simulink model "slider_mode_controller_kalman_filter_sim_18"  (R2022a)
settings: Solver=ode5  StartTime=0.0  StopTime=700  RelTol=1e-3  EnableMultiTasking=on
undefined symbols (not defined in the file): sim_output_sample_time, sim_r
libraries: simulink x1
settings Model: Creator=wolfgang  LastModifiedBy=Alghisi
settings Model: ModifiedHistory=|
  | Created an adjusted empty Simulink diagram for the lab assignments
  | in the course R0002E
settings SolverCC: AlgebraicLoopSolver=TrustRegion
settings DataIOCC: SaveFormat=Array  SignalLoggingSaveFormat=ModelDataLogs  SaveOutput=off  SignalLogging=off  DSMLogging=off  SaveTime=off  ReturnWorkspaceOutputs=off
settings OptimizationCC: ExpressionDepthLimit=2147483647  LifeSpan=inf
settings DebuggingCC: UnderspecifiedInitializationDetection=Classic  MergeDetectMultiDrivingBlocksExec=none  SolverPrmCheckMsg=warning  FcnCallInpInsideContextMsg=warning  UnconnectedInputMsg=warning  UnconnectedOutputMsg=warning  UnconnectedLineMsg=warning  StateNameClashWarn=warning  SFUnexpectedBacktrackingDiag=warning  SFNoUnconditionalDefaultTransitionDiag=warning  SFExecutionAtInitializationDiag=none  SFMachineParentedDataDiag=warning  ArithmeticOperatorsInVariantConditions=warning
settings HardwareCC: ProdBitPerPointer=32  ProdBitPerSizeT=32  ProdBitPerPtrDiffT=32  ProdLargestAtomicFloat=None  ProdIntDivRoundTo=Undefined  ProdEndianess=Unspecified  ProdWordSize=32  ProdHWDeviceType=32-bit Generic
settings ModelReferenceCC: PropagateSignalLabelsOutOfModel=off
settings SFSimCC: SimUseLocalCustomCode=off  CustomCodeUndefinedFunction=UseInterfaceOnly
settings RTWCC: RTWUseLocalCustomCode=off
settings CodeAppCC: StateflowObjectComments=on
settings GRTTargetCC: TargetLangStandard=C89/C90 (ANSI)
settings ConfigComp: CovMetricSettings=dw  CovSaveCumulativeToWorkspaceVar=on  CovSaveSingleToWorkspaceVar=on  CovExternalEMLEnable=off  CovSFcnEnable=off

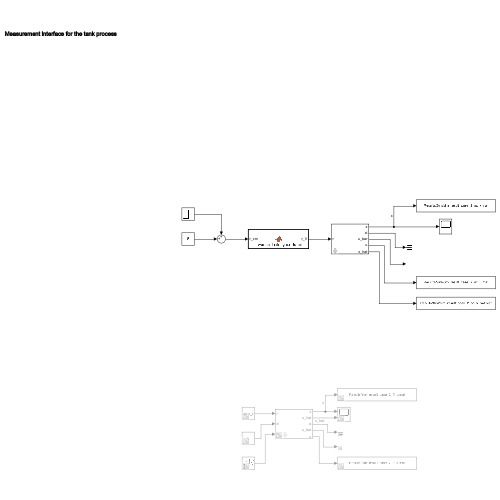
[thumbnail: Simulink's stored preview of the top-level diagram]
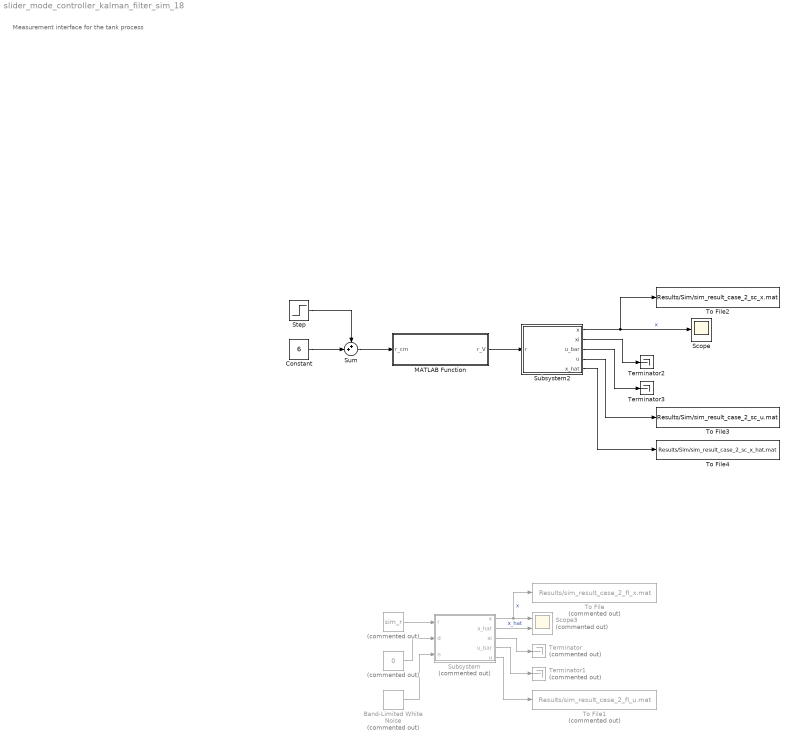
== system slider_mode_controller_kalman_filter_sim_18 ==
  note: Measurement interface for the tank process
  "  " : Constant  Commented=on  Value=0
  "      " : Constant  Commented=on  Value=sim_r
  Band-Limited White Noise : simulink/Sources/Band-Limited White Noise  Commented=on  Cov=0.00001  Ts=0.1  seed=[23341]
  Constant : Constant  Value=6
  MATLAB Function : MATLAB Function  TreatAsAtomicUnit=on
  Scope : Scope
  Scope3 : Scope  Commented=on  NumInputPorts=2
  Step : Step  Time=300  After=2  SampleTime=0
  Subsystem : Subsystem  Commented=on  mask{init_state_param=[8;8], Integrator_gain_param=0.01}
      mask prompts: init_state_param "Initial state"; Integrator_gain_param "Integrator gain"
  Subsystem2 : Subsystem  mask{p1_param=0.1, p2_param=0.2, epsi_param=0.5, mu_param=0.2}
      mask prompts: p1_param "p1"; p2_param "p2"; epsi_param "epsi"; mu_param "mu"
  Sum : Sum  Inputs=++|
  Terminator : Terminator  Commented=on
  Terminator1 : Terminator  Commented=on
  Terminator2 : Terminator
  Terminator3 : Terminator
  To File : ToFile  Commented=on  Filename=Results/sim_result_case_2_fl_x.mat  MatrixName=sim_result_case_2_fl_x  SaveFormat=Timeseries  SampleTime=sim_output_sample_time
  To File1 : ToFile  Commented=on  Filename=Results/sim_result_case_2_fl_u.mat  MatrixName=sim_result_case_2_fl_u  SaveFormat=Timeseries  SampleTime=sim_output_sample_time
  To File2 : ToFile  Filename=Results/Sim/sim_result_case_2_sc_x.mat  MatrixName=sim_result_case_2_sc_x  SaveFormat=Timeseries  SampleTime=0.02
  To File3 : ToFile  Filename=Results/Sim/sim_result_case_2_sc_u.mat  MatrixName=sim_result_case_2_sc_u  SaveFormat=Timeseries  SampleTime=0.02
  To File4 : ToFile  Filename=Results/Sim/sim_result_case_2_sc_x_hat.mat  MatrixName=sim_result_case_2_sc_x_hat  SaveFormat=Timeseries  SampleTime=0.02
  wires:
  Subsystem/2(x_hat) -> Scope3/2  "x_hat"
  "  "/1 -> Subsystem/2(d)
  "      "/1 -> Subsystem/1(r)
  Band-Limited White Noise/1 -> Subsystem/3(n)
  Subsystem/1(x) -> Scope3/1, To File/1  "x"
  Subsystem/3(xi) -> Terminator/1
  Subsystem/4(u_bar) -> Terminator1/1
  Subsystem/5(u) -> To File1/1
  Subsystem2/2(xi) -> Terminator2/1
  MATLAB Function/1(r_V) -> Subsystem2/1(r)
  Subsystem2/3(u_bar) -> Terminator3/1
  Subsystem2/4(u) -> To File3/1
  Subsystem2/1(x) -> Scope/1, To File2/1  "x"
  Constant/1 -> Sum/2
  Sum/1 -> MATLAB Function/1(r_cm)
  Step/1 -> Sum/1
  Subsystem2/5(x_hat) -> To File4/1

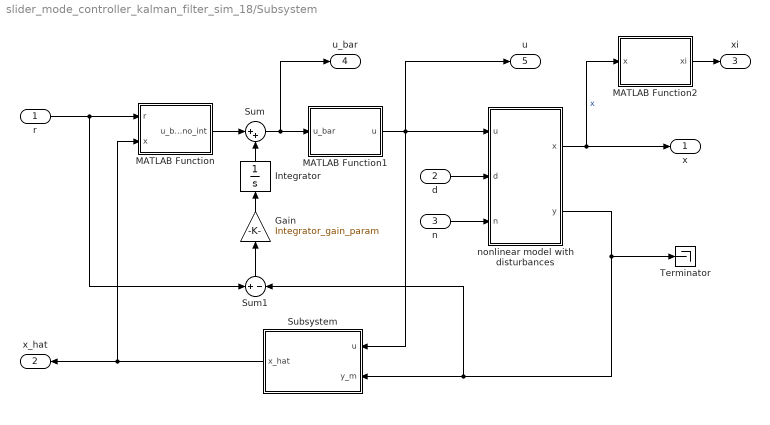
== system slider_mode_controller_kalman_filter_sim_18/Subsystem ==
  r : Inport
  d : Inport  Port=2
  n : Inport  Port=3
  Gain : Gain  Gain=Integrator_gain_param
  Integrator : Integrator
  MATLAB Function : MATLAB Function  TreatAsAtomicUnit=on
  MATLAB Function1 : MATLAB Function  TreatAsAtomicUnit=on
  MATLAB Function2 : MATLAB Function  TreatAsAtomicUnit=on
  Subsystem : Subsystem
  Sum : Sum  Inputs=|++
  Sum1 : Sum  Inputs=+-
  Terminator : Terminator
  nonlinear model with disturbances : Subsystem
  x : Outport
  x_hat : Outport  Port=2
  xi : Outport  Port=3
  u_bar : Outport  Port=4
  u : Outport  Port=5
  wires:
  Sum1/1 -> Gain/1
  Gain/1 -> Integrator/1
  Integrator/1 -> Sum/2
  MATLAB Function/1(u_bar_no_int) -> Sum/1
  Sum/1 -> MATLAB Function1/1(u_bar), u_bar/1
  nonlinear model with disturbances/2(y) -> Terminator/1, Subsystem/2(y_m), Sum1/2
  MATLAB Function1/1(u) -> Subsystem/1(u), nonlinear model with disturbances/1(u), u/1
  nonlinear model with disturbances/1(x) -> MATLAB Function2/1(x), x/1  "x"
  d/1 -> nonlinear model with disturbances/2(d)
  n/1 -> nonlinear model with disturbances/3(n)
  MATLAB Function2/1(xi) -> xi/1
  r/1 -> Sum1/1, MATLAB Function/1(r)
  Subsystem/1(x_hat) -> x_hat/1, MATLAB Function/2(x)

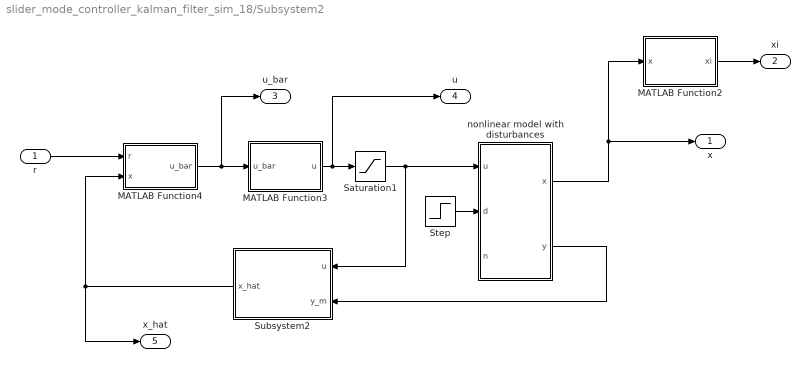
== system slider_mode_controller_kalman_filter_sim_18/Subsystem2 ==
  r : Inport
  MATLAB Function2 : MATLAB Function  TreatAsAtomicUnit=on
  MATLAB Function3 : MATLAB Function  TreatAsAtomicUnit=on
  MATLAB Function4 : MATLAB Function  TreatAsAtomicUnit=on
  Saturation1 : Saturate  UpperLimit=10  LowerLimit=0
  Step : Step  Time=500  After=0.05  SampleTime=0
  Subsystem2 : Subsystem
  nonlinear model with disturbances : Subsystem
  x : Outport
  xi : Outport  Port=2
  u_bar : Outport  Port=3
  u : Outport  Port=4
  x_hat : Outport  Port=5
  wires:
  MATLAB Function2/1(xi) -> xi/1
  nonlinear model with disturbances/1(x) -> x/1, MATLAB Function2/1(x)
  MATLAB Function4/1(u_bar) -> MATLAB Function3/1(u_bar), u_bar/1
  r/1 -> MATLAB Function4/1(r)
  MATLAB Function3/1(u) -> u/1, Saturation1/1
  nonlinear model with disturbances/2(y) -> Subsystem2/2(y_m)
  Subsystem2/1(x_hat) -> x_hat/1, MATLAB Function4/2(x)
  Step/1 -> nonlinear model with disturbances/2(d)
  Saturation1/1 -> Subsystem2/1(u), nonlinear model with disturbances/1(u)

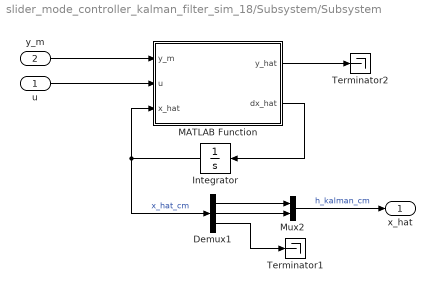
== system slider_mode_controller_kalman_filter_sim_18/Subsystem/Subsystem ==
  u : Inport
  y_m : Inport  Port=2
  Demux1 : Demux  Outputs=3
  Integrator : Integrator  InitialCondition=[init_state_param;0]
  MATLAB Function : MATLAB Function  TreatAsAtomicUnit=on
  Mux2 : Mux  Inputs=2
  Terminator1 : Terminator
  Terminator2 : Terminator
  x_hat : Outport
  wires:
  Mux2/1 -> x_hat/1  "h_kalman_cm"
  MATLAB Function/2(dx_hat) -> Integrator/1
  MATLAB Function/1(y_hat) -> Terminator2/1
  y_m/1 -> MATLAB Function/1(y_m)
  u/1 -> MATLAB Function/2(u)
  Integrator/1 -> MATLAB Function/3(x_hat), Demux1/1  "x_hat_cm"
  Demux1/2 -> Mux2/2
  Demux1/1 -> Mux2/1
  Demux1/3 -> Terminator1/1

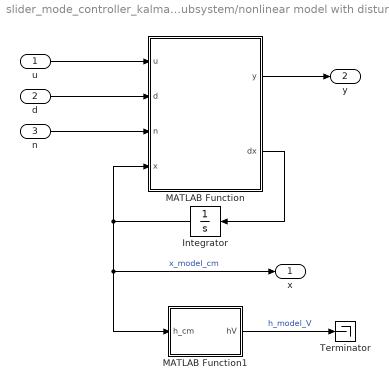
== system slider_mode_controller_kalman_filter_sim_18/Subsystem/nonlinear model with disturbances ==
  u : Inport
  d : Inport  Port=2
  n : Inport  Port=3
  Integrator : Integrator  InitialCondition=init_state_param
  MATLAB Function : MATLAB Function  TreatAsAtomicUnit=on
  MATLAB Function1 : MATLAB Function  TreatAsAtomicUnit=on
  Terminator : Terminator
  x : Outport
  y : Outport  Port=2
  wires:
  u/1 -> MATLAB Function/1(u)
  Integrator/1 -> x/1, MATLAB Function1/1(h_cm), MATLAB Function/4(x)  "x_model_cm"
  MATLAB Function/2(dx) -> Integrator/1
  d/1 -> MATLAB Function/2(d)
  MATLAB Function1/1(hV) -> Terminator/1  "h_model_V"
  n/1 -> MATLAB Function/3(n)
  MATLAB Function/1(y) -> y/1

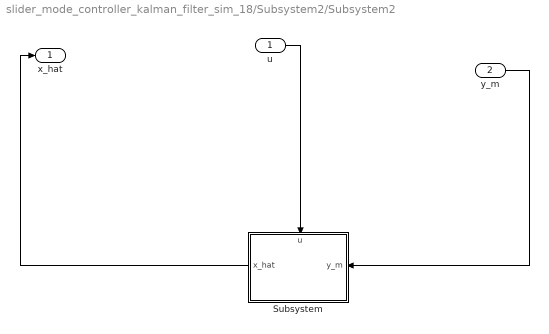
== system slider_mode_controller_kalman_filter_sim_18/Subsystem2/Subsystem2 ==
  u : Inport
  y_m : Inport  Port=2
  Subsystem : Subsystem
      settings: PortSchema="{\"entries\":[{\"content\":{\"sides\":[{\"content\":{\"connectorIds\":[\"In1\"]},\"type\":\"ConnectorPlacement.EquallySpacedRectSide\",\"uuid\":\"86b77032-109f-4880-bda9-8eff247771ee\"},{\"content\":{\"connectorIds\":[\"Out1\"],\"side\":\"RIGHT\"},\"type\":\"ConnectorPlacement.EquallySpacedRectSide\",\"uuid\":\"f6e7be45-afa8-48cd-9ff2-8e89d09ed8f0\"},{\"content\":{\"connectorIds\":[\"In2\"],\"side\":\"TOP\"},\"type\":\"ConnectorPlacement.EquallySpacedRectSide\",\"uuid\":\"c04b745c-f514-4b60-a02c-bc4ff2757180\"}]},\"type\":\"ConnectorPlacement.EquallySpacedConnector\",\"uuid\":\"f26e49cc-92a6-4411-ab59-9b13f847a501\"}],\"packageUris\":[\"http://schema.mathworks.com/mf0/Connector/19700101\"],\"version\":\"1.0\"}"
  x_hat : Outport
  wires:
  Subsystem/1(x_hat) -> x_hat/1
  y_m/1 -> Subsystem/1(y_m)
  u/1 -> Subsystem/2(u)

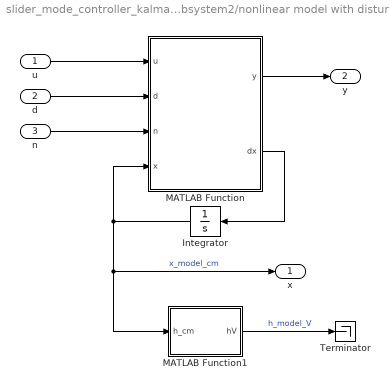
== system slider_mode_controller_kalman_filter_sim_18/Subsystem2/nonlinear model with disturbances ==
  u : Inport
  d : Inport  Port=2
  n : Inport  Port=3
  Integrator : Integrator  InitialCondition=[0;0]
  MATLAB Function : MATLAB Function  TreatAsAtomicUnit=on
  MATLAB Function1 : MATLAB Function  TreatAsAtomicUnit=on
  Terminator : Terminator
  x : Outport
  y : Outport  Port=2
  wires:
  MATLAB Function/1(y) -> y/1
  n/1 -> MATLAB Function/3(n)
  MATLAB Function1/1(hV) -> Terminator/1  "h_model_V"
  d/1 -> MATLAB Function/2(d)
  MATLAB Function/2(dx) -> Integrator/1
  Integrator/1 -> MATLAB Function/4(x), MATLAB Function1/1(h_cm), x/1  "x_model_cm"
  u/1 -> MATLAB Function/1(u)

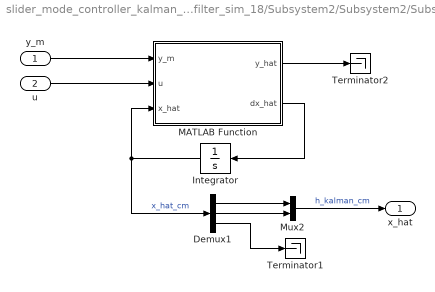
== system slider_mode_controller_kalman_filter_sim_18/Subsystem2/Subsystem2/Subsystem ==
  y_m : Inport
  u : Inport  Port=2
  Demux1 : Demux  Outputs=3
  Integrator : Integrator  InitialCondition=[0;0;0]
  MATLAB Function : MATLAB Function  TreatAsAtomicUnit=on
  Mux2 : Mux  Inputs=2
  Terminator1 : Terminator
  Terminator2 : Terminator
  x_hat : Outport
  wires:
  Mux2/1 -> x_hat/1  "h_kalman_cm"
  MATLAB Function/2(dx_hat) -> Integrator/1
  MATLAB Function/1(y_hat) -> Terminator2/1
  y_m/1 -> MATLAB Function/1(y_m)
  u/1 -> MATLAB Function/2(u)
  Integrator/1 -> MATLAB Function/3(x_hat), Demux1/1  "x_hat_cm"
  Demux1/2 -> Mux2/2
  Demux1/1 -> Mux2/1
  Demux1/3 -> Terminator1/1

== matlab function slider_mode_controller_kalman_filter_sim_18/Subsystem2/MATLAB Function3 ==
  data: u_bar input; u output
function u = pm1(u_bar)

u = u_bar.*3.277899884284337e-1-u_bar.^2.*9.88758313621772e-3+u_bar.^3.*1.567756031883916e-4-2.914041336753123;

end

== matlab function slider_mode_controller_kalman_filter_sim_18/Subsystem2/MATLAB Function4 ==
  data: r input; u_bar output; x input; mu_param parameter; p1_param parameter; p2_param parameter; epsi_param parameter
function u_bar = fcn(r,x, mu_param, p1_param, p2_param, epsi_param)

mu = mu_param;
epsi = epsi_param;
p1 = p1_param;
p2 = p2_param;

x1=x(1);
x2=x(2);

u_bar = ((p2.*(sqrt(x1.*5.0+1.6e+1).*7.609042393596842e-2-sqrt(x2.*5.0+1.6e+1).*7.609042393596842e-2).*1.0./sqrt(abs(p1).^2+abs(p2).^2)+p1.*1.0./sqrt(x1.*5.0+1.6e+1).*1.0./sqrt(x2.*5.0+1.6e+1).*(x1.*2.7795e+4+8.8944e+4).*1.0./sqrt(abs(p1).^2+abs(p2).^2).*3.491988616282361e-6).*sqrt(x1.*5.0+1.6e+1).*sqrt(abs(p1).^2+abs(p2).^2).*(-1.734778086018821e+2))./p1-(mu.*sqrt(x1.*5.0+1.6e+1).*sqrt(abs(p1).^2+abs(p2).^2).*min([1.0,max([-1.0,(p1.*(sqrt(x1.*1.962e+3+6.2784e+3).*3.841187477910597e-3-sqrt(x2.*1.962e+3+6.2784e+3).*3.841187477910597e-3)-p2.*(r-x2.*7.456422751238219e-1+1.648066384406454))./epsi],[],2,'omitnan')],[],2,'omitnan').*1.734778086018821e+2)./p1;


end

== matlab function slider_mode_controller_kalman_filter_sim_18/Subsystem2/nonlinear model with disturbances/MATLAB Function1 ==
  data: h_cm input; hV output
function hV = g(h_cm)

hV = h_cm*7.456422751238219e-1 - 1.648066384406454;

== matlab function slider_mode_controller_kalman_filter_sim_18/MATLAB Function ==
  data: r_cm input; r_V output
function r_V = i_wanna_hold_your_hand(r_cm)

z = r_cm;

r_V = 0.74564227512382186269235262443544*z - 1.6480663844064573630987524666125;

end

== matlab function slider_mode_controller_kalman_filter_sim_18/Subsystem2/nonlinear model with disturbances/MATLAB Function ==
  data: y output; u input; dx output; d input; n input; x input
function [y,dx] = nonlinear_model(u,d,n,x)

x1 = x(1);
x2 = x(2);

y = x2.*7.456422751238219e-1 + n -1.648066384406454;

dx = [+u.*2.81859116712929e-1-(d.*sqrt(x1.*1.962e+3+6.2784e+3))./3.3e+1-sqrt(x1.*1.962e+3+6.2784e+3).*5.151515151515152e-3-u.^2.*2.476601319356692e-2+u.^3.*8.808489605974731e-4+3.751072019731428e-1;sqrt(x1.*1.962e+3+6.2784e+3).*5.151515151515152e-3-sqrt(x2.*1.962e+3+6.2784e+3).*5.151515151515152e-3];

end

== matlab function slider_mode_controller_kalman_filter_sim_18/Subsystem/Subsystem/MATLAB Function ==
  data: y_hat output; y_m input; u input; x_hat input; dx_hat output
function [y_hat,dx_hat]  = kalman_filter(y_m,u,x_hat)

x1_hat = x_hat(1);
x2_hat = x_hat(2);
x3_hat = x_hat(3);

dx_hat = [x1_hat.*(-3.409145021215564e-2)-x2_hat.*4.707003693403074e-1+u.*2.098905560223644e-1+y_m.*6.312683508484582e-1-sqrt(5.0).*sqrt(7.63e+2).*x3_hat.*(4.0./5.5e+1)+9.799223895936307e-1;
    x1_hat.*3.409145021215564e-2-x2_hat.*1.823621215877479e-1+y_m.*1.98849604323964e-1+3.277173484388494e-1;x2_hat.*7.456422751238219e-3-y_m./1.0e+2-1.648066384406454e-2];

y_hat = x2_hat.*7.456422751238219e-1-1.648066384406454;

end

== matlab function slider_mode_controller_kalman_filter_sim_18/Subsystem2/Subsystem2/Subsystem/MATLAB Function ==
  data: y_hat output; y_m input; u input; x_hat input; dx_hat output
function [y_hat,dx_hat]  = kalman_filter(y_m,u,x_hat)

x1_hat = x_hat(1);
x2_hat = x_hat(2);
x3_hat = x_hat(3);

dx_hat = [x1_hat.*(-3.409145021215564e-2)-x2_hat.*4.707003693403074e-1+u.*2.098905560223644e-1+y_m.*6.312683508484582e-1-sqrt(5.0).*sqrt(7.63e+2).*x3_hat.*(4.0./5.5e+1)+9.799223895936307e-1;
    x1_hat.*3.409145021215564e-2-x2_hat.*1.823621215877479e-1+y_m.*1.98849604323964e-1+3.277173484388494e-1;x2_hat.*7.456422751238219e-3-y_m./1.0e+2-1.648066384406454e-2];

y_hat = x2_hat.*7.456422751238219e-1-1.648066384406454;

end

== matlab function slider_mode_controller_kalman_filter_sim_18/Subsystem2/MATLAB Function2 ==
  data: x input; xi output
function xi = T(x)

x1 = x(1);
x2 = x(2);

xi = [x2.*7.456422751238219e-1-1.648066384406454;sqrt(x1.*1.962e+3+6.2784e+3).*3.841187477910597e-3-sqrt(x2.*1.962e+3+6.2784e+3).*3.841187477910597e-3];

end

== matlab function slider_mode_controller_kalman_filter_sim_18/Subsystem/MATLAB Function ==
  data: r input; x input; u_bar_no_int output
function u_bar_no_int = k(r,x)

x1 = x(1);
x2 = x(2);

u_bar_no_int = sqrt(x1.*1.962e+3+6.2784e+3).*(r.*(3.0./8.0e+2)-x2.*2.796158531714332e-3+1.0./sqrt(x2.*1.962e+3+6.2784e+3).*(sqrt(x1.*1.962e+3+6.2784e+3).*5.151515151515152e-3-sqrt(x2.*1.962e+3+6.2784e+3).*5.151515151515152e-3).*3.768204915830296-sqrt(x1.*1.962e+3+6.2784e+3).*4.801484347388247e-4+sqrt(x2.*1.962e+3+6.2784e+3).*4.801484347388247e-4+2.559221365943785e-2).*8.757485523509194;

end

== matlab function slider_mode_controller_kalman_filter_sim_18/Subsystem/MATLAB Function1 ==
  data: u_bar input; u output
function u = pm1(u_bar)

u = u_bar.*3.277899884284337e-1-u_bar.^2.*9.88758313621772e-3+u_bar.^3.*1.567756031883916e-4-2.914041336753123;

end

== matlab function slider_mode_controller_kalman_filter_sim_18/Subsystem/MATLAB Function2 ==
  data: x input; xi output
function xi = T(x)

x1 = x(1);
x2 = x(2);

xi = [x2.*7.456422751238219e-1-1.648066384406454;sqrt(x1.*1.962e+3+6.2784e+3).*3.841187477910597e-3-sqrt(x2.*1.962e+3+6.2784e+3).*3.841187477910597e-3];

end

== matlab function slider_mode_controller_kalman_filter_sim_18/Subsystem/nonlinear model with disturbances/MATLAB Function ==
  data: y output; u input; dx output; d input; n input; x input
function [y,dx] = nonlinear_model(u,d,n,x)

x1 = x(1);
x2 = x(2);

y = x2.*7.456422751238219e-1 + n -1.648066384406454;

dx = [+u.*2.81859116712929e-1-(d.*sqrt(x1.*1.962e+3+6.2784e+3))./3.3e+1-sqrt(x1.*1.962e+3+6.2784e+3).*5.151515151515152e-3-u.^2.*2.476601319356692e-2+u.^3.*8.808489605974731e-4+3.751072019731428e-1;sqrt(x1.*1.962e+3+6.2784e+3).*5.151515151515152e-3-sqrt(x2.*1.962e+3+6.2784e+3).*5.151515151515152e-3];

end

== matlab function slider_mode_controller_kalman_filter_sim_18/Subsystem/nonlinear model with disturbances/MATLAB Function1 ==
  data: h_cm input; hV output
function hV = g(h_cm)

hV = h_cm*7.456422751238219e-1 - 1.648066384406454;
